simulink model "SWC_HALIN_CDD_type"  (R2021b)
settings: Solver=FixedStepDiscrete  StartTime=0.0  StopTime=10.0  FixedStep=0.005  RelTol=1e-3
values from neighbouring files (symbols this model uses):
  C_TASK_5MS_S = (	C_TICK_TIME_S      	)    [vcu_local_hdr.m]    (also in vcu_local_hdrTA2.m)
  DIDLen_APSFunConfig = uint16(16)    [vcu_local_hdr.m]
  DIDLen_AutoLock = uint16(1)    [vcu_local_hdr.m]
  DIDLen_AutoWipHSpdEN = uint16(1)    [vcu_local_hdr.m]
  DIDLen_DKCKey = uint16(8)    [vcu_local_hdr.m]
  DIDLen_DRLDis = uint16(1)    [vcu_local_hdr.m]
  DIDLen_DynoMode = uint16(1)    [vcu_local_hdr.m]
  DIDLen_FMHTimer = uint16(1)    [vcu_local_hdr.m]
  DIDLen_TireSize = uint16(16)    [vcu_local_hdr.m]
  DIDLen_TurnLampFLThreCurr = uint16(1)    [vcu_local_hdr.m]
  DIDLen_TurnLampFRThreCurr = uint16(1)    [vcu_local_hdr.m]
  DIDLen_TurnLampRLThreCurr = uint16(1)    [vcu_local_hdr.m]
  DIDLen_TurnLampRRThreCurr = uint16(1)    [vcu_local_hdr.m]
  DIDLen_USSConfig = uint16(16)    [vcu_local_hdr.m]
  DIDLen_WipRLSCmdCutFilter = uint16(1)    [vcu_local_hdr.m]
  DIDLen_WipRLSCmdHoldFilter = uint16(1)    [vcu_local_hdr.m]
  DIDLen_XWDMode = uint16(1)    [vcu_local_hdr.m]
  DIDNum_APSFunConfig = uint16(0x0903)    [vcu_local_hdr.m]
  DIDNum_AutoLock = uint16(0x0306)    [vcu_local_hdr.m]
  DIDNum_AutoWipHSpdEN = uint16(0x0308)    [vcu_local_hdr.m]
  DIDNum_DKCKey = uint16(0x0202)    [vcu_local_hdr.m]
  DIDNum_DRLDis = uint16(0x0307)    [vcu_local_hdr.m]
  DIDNum_DynoMode = uint16(0x0203)    [vcu_local_hdr.m]
  DIDNum_FMHTimer = uint16(0x0305)    [vcu_local_hdr.m]
  DIDNum_TireSize = uint16(0x0902)    [vcu_local_hdr.m]
  DIDNum_TurnLampFLThreCurr = uint16(0x0303)    [vcu_local_hdr.m]
  DIDNum_TurnLampFRThreCurr = uint16(0x0301)    [vcu_local_hdr.m]
  DIDNum_TurnLampRLThreCurr = uint16(0x0304)    [vcu_local_hdr.m]
  DIDNum_TurnLampRRThreCurr = uint16(0x0302)    [vcu_local_hdr.m]
  DIDNum_USSConfig = uint16(0x0901)    [vcu_local_hdr.m]
  DIDNum_WipRLSCmdCutFilter = uint16(0x030A)    [vcu_local_hdr.m]
  DIDNum_WipRLSCmdHoldFilter = uint16(0x0309)    [vcu_local_hdr.m]
  DIDNum_XWDMode = uint16(0x0201)    [vcu_local_hdr.m]
  ENUM_DRIVETRAIN_AWD = uint8(  2  )    [vcu_local_hdr.m]
  ENUM_DRIVETRAIN_FWD = uint8(  1  )    [vcu_local_hdr.m]
  ENUM_DRIVETRAIN_RWD = uint8(  0  )    [vcu_local_hdr.m]
  ENUM_REGENLEVEL_LV1 = uint8(  1  )    [vcu_local_hdr.m]
  ENUM_REGENLEVEL_LV2 = uint8(  2  )    [vcu_local_hdr.m]
  ENUM_REGENLEVEL_LV3 = uint8(  3  )    [vcu_local_hdr.m]
  ENUM_REGENLEVEL_LV4 = uint8(  4  )    [vcu_local_hdr.m]
  ENUM_REGENLEVEL_LV5 = uint8(  5  )    [vcu_local_hdr.m]
  ENUM_REGENLEVEL_OPD = uint8(  6  )    [vcu_local_hdr.m]
  ENUM_TPMSSTA_FAT = uint8(  8  )    [vcu_local_hdr.m]
  ENUM_TPMSSTA_LOWBATTERY = uint8(  2  )    [vcu_local_hdr.m]
  ENUM_TPMSSTA_TRIGGER = uint8(  4  )    [vcu_local_hdr.m]
  FALSE = boolean( 0 )    [vcu_local_hdr.m]    (also in vcu_local_hdrTA2.m)
  ONE_INT = uint8(1)    [vcu_local_hdr.m]    (also in vcu_local_hdrTA2.m)
  TRUE = boolean( 1 )    [vcu_local_hdr.m]    (also in vcu_local_hdrTA2.m)
  ZERO_FLOAT = single(0)    [vcu_local_hdr.m]    (also in vcu_local_hdrTA2.m)
  ZERO_INT = uint8(0)    [vcu_local_hdr.m]    (also in vcu_local_hdrTA2.m)
undefined symbols (not defined in the file or in its folder): KHAL_CANBusOffDebounce_s, KHAL_DefaultRegenMode_enum, KHAL_DKCDecryptEnable_flg_ovrdflg, KHAL_DKCDecryptEnable_flg_ovrdval, KHAL_RandomNumberY1_enum, KHAL_RandomNumberY2_enum, KHAL_RandomNumberY_ovrdflg, KHAL_TPMSRESBUTT_flg_ovrdflg, KHAL_TPMSRESBUTT_flg_ovrdval, KINP_ReadVinCode_flg, R_NVMReadCDD_Inner_NVM_ReadOperation
libraries: simulink x112, hcu_lib x23, hdlsllib x8
(part 1 of 7)
settings Model: DataDictionary=APPTypes.sldd  Creator=FVT22063  LastModifiedBy=FVT23033
settings DataIOCC: SaveFormat=StructureWithTime
settings OptimizationCC: DefaultParameterBehavior=Inlined  EnhancedBackFolding=on  PassReuseOutputArgsAs=Individual arguments  ZeroExternalMemoryAtStartup=off  ZeroInternalMemoryAtStartup=off  OptimizeBlockOrder=speed  DifferentSizesBufferReuse=on  OptimizationCustomize=off  EfficientTunableParamExpr=on
settings DebuggingCC: ParameterTunabilityLossMsg=error
settings HardwareCC: ProdBitPerPointer=32  ProdBitPerSizeT=32  ProdBitPerPtrDiffT=32  ProdLargestAtomicInteger=Long  ProdLargestAtomicFloat=Double  ProdWordSize=32  ProdLongLongMode=on  ProdHWDeviceType=ARM Compatible->ARM Cortex-M
settings ModelReferenceCC: ModelReferenceNumInstancesAllowed=Single
settings SFSimCC: MATLABDynamicMemAlloc=off
settings RTWCC: Description=AUTOSAR  SystemTargetFile=autosar.tlc  GenCodeOnly=on  TemplateMakefile=ert_default_tmf  PortableWordSizes=on
settings CodeAppCC: ForceParamTrailComments=on  IgnoreCustomStorageClasses=off  OperatorAnnotations=on  SimulinkDataObjDesc=on  SFDataObjDesc=on  InsertBlockDesc=on
settings STFCustomTargetCC: TargetLangStandard=C99 (ISO)  MultiwordLength=256  ParMdlRefBuildCompliant=on  CompOptLevelCompliant=on  IncludeMdlTerminateFcn=off  CombineOutputUpdateFcns=on  SuppressErrorStatus=on  ERTCustomFileBanners=on  SupportNonFinite=off  SupportComplex=off  SupportContinuousTime=off  SupportNonInlinedSFcns=off  RemoveResetFunc=on  MATLABClassNameForMDSCustomization=Simulink.SoftwareTarget.ERTCustomization  AutosarCompliant=on  GRTInterface=off  UseToolchainInfoCompliant=on  LookupTableObjectStructAxisOrder=2,1,3,4,...  LUTObjectStructOrderEvenSpacing=Size,Table,Breakpoints  SystemTargetFile=autosar.tlc
settings ERTTargetCC: TargetLangStandard=C99 (ISO)  ConcurrentExecutionCompliant=off  IncludeMdlTerminateFcn=off  SuppressErrorStatus=on  SupportNonFinite=off  SupportComplex=off  ModelStepFunctionPrototypeControlCompliant=off  CPPClassGenCompliant=off  AutosarCompliant=on  LookupTableObjectStructAxisOrder=2,1,3,4,...  LUTObjectStructOrderEvenSpacing=Size,Table,Breakpoints  GenerateASAP2=on  InlinedParameterPlacement=NonHierarchical  ERTCustomFileTemplate=example_file_process.tlc  ConvertIfToSwitch=off  SuppressUnreachableDefaultCases=off  BooleanTrueId=true_MatlabRTW  BooleanFalseId=false_MatlabRTW

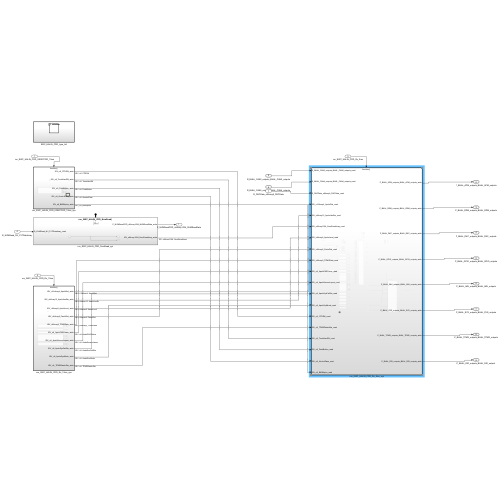
[thumbnail: Simulink's stored preview of the top-level diagram]
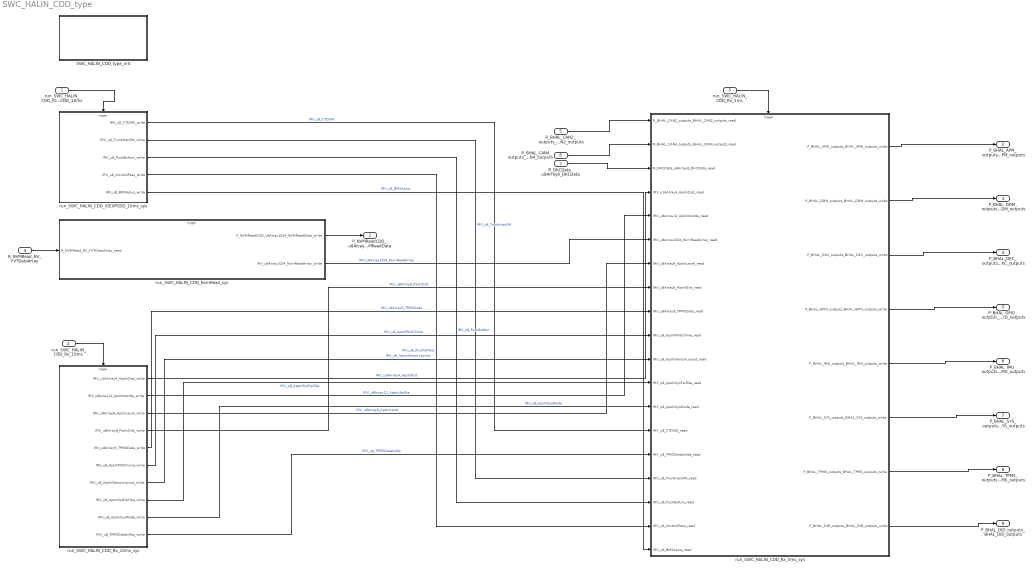
== system SWC_HALIN_CDD_type ==
  run_SWC_HALIN_CDD_IOEXPCDD_10ms : Inport  SampleTime=0.01  OutputFunctionCall=on
  run_SWC_HALIN_CDD_Rx_10ms : Inport  Port=2  SampleTime=0.01  OutputFunctionCall=on
  run_SWC_HALIN_CDD_Rx_5ms : Inport  Port=3  SampleTime=0.005  OutputFunctionCall=on
  R_NVMRead_NV_FVTDataArray : Inport  Port=4  OutDataTypeStr=uint8  PortDimensions=1024
  R_BHAL_CAN2_outputs_BHAL_CAN2_outputs : Inport  Port=5  OutDataTypeStr=Bus: BHAL_CAN2_outputs  PortDimensions=1  BusOutputAsStruct=on
  R_BHAL_CAN4_outputs_BHAL_CAN4_outputs : Inport  Port=6  OutDataTypeStr=Bus: BHAL_CAN4_outputs  PortDimensions=1  BusOutputAsStruct=on
  R_DKCData_u8Array8_DKCData : Inport  Port=7  OutDataTypeStr=uint8  PortDimensions=8
  SWC_HALIN_CDD_type_Init : Subsystem
  run_SWC_HALIN_CDD_IOEXPCDD_10ms_sys : Subsystem
  run_SWC_HALIN_CDD_NvmRead_sys : Subsystem
  run_SWC_HALIN_CDD_Rx_10ms_sys : Subsystem
  run_SWC_HALIN_CDD_Rx_5ms_sys : Subsystem
  P_NVMReadCDD_u8Array1024_NVMReadData : Outport  OutDataTypeStr=uint8  PortDimensions=1024
  P_BHAL_APM_outputs_BHAL_APM_outputs : Outport  Port=2  OutDataTypeStr=Bus: BHAL_APM_outputs  PortDimensions=1  BusOutputAsStruct=on
  P_BHAL_DDM_outputs_BHAL_DDM_outputs : Outport  Port=3  OutDataTypeStr=Bus: BHAL_DDM_outputs  PortDimensions=1  BusOutputAsStruct=on
  P_BHAL_DKC_outputs_BHAL_DKC_outputs : Outport  Port=4  OutDataTypeStr=Bus: BHAL_DKC_outputs  PortDimensions=1  BusOutputAsStruct=on
  P_BHAL_GPIO_outputs_BHAL_GPIO_outputs : Outport  Port=5  OutDataTypeStr=Bus: BHAL_GPIO_outputs  PortDimensions=1  BusOutputAsStruct=on
  P_BHAL_IMU_outputs_BHAL_IMU_outputs : Outport  Port=6  OutDataTypeStr=Bus: BHAL_IMU_outputs  PortDimensions=1  BusOutputAsStruct=on
  P_BHAL_SYS_outputs_BHAL_SYS_outputs : Outport  Port=7  OutDataTypeStr=Bus: BHAL_SYS_outputs  PortDimensions=1  BusOutputAsStruct=on
  P_BHAL_TPMS_outputs_BHAL_TPMS_outputs : Outport  Port=8  OutDataTypeStr=Bus: BHAL_TPMS_outputs  PortDimensions=1  BusOutputAsStruct=on
  P_BHAL_DID_outputs_BHAL_DID_outputs : Outport  Port=9  OutDataTypeStr=Bus: BHAL_DID_outputs  PortDimensions=1  BusOutputAsStruct=on
  wires:
  R_NVMRead_NV_FVTDataArray/1 -> run_SWC_HALIN_CDD_NvmRead_sys/1(R_NVMRead_NV_FVTDataArray_read)
  run_SWC_HALIN_CDD_NvmRead_sys/1(P_NVMReadCDD_u8Array1024_NVMReadData_write) -> P_NVMReadCDD_u8Array1024_NVMReadData/1
  R_BHAL_CAN2_outputs_BHAL_CAN2_outputs/1 -> run_SWC_HALIN_CDD_Rx_5ms_sys/1(R_BHAL_CAN2_outputs_BHAL_CAN2_outputs_read)
  R_BHAL_CAN4_outputs_BHAL_CAN4_outputs/1 -> run_SWC_HALIN_CDD_Rx_5ms_sys/2(R_BHAL_CAN4_outputs_BHAL_CAN4_outputs_read)
  R_DKCData_u8Array8_DKCData/1 -> run_SWC_HALIN_CDD_Rx_5ms_sys/3(R_DKCData_u8Array8_DKCData_read)
  run_SWC_HALIN_CDD_Rx_5ms_sys/1(P_BHAL_APM_outputs_BHAL_APM_outputs_write) -> P_BHAL_APM_outputs_BHAL_APM_outputs/1
  run_SWC_HALIN_CDD_Rx_5ms_sys/2(P_BHAL_DDM_outputs_BHAL_DDM_outputs_write) -> P_BHAL_DDM_outputs_BHAL_DDM_outputs/1
  run_SWC_HALIN_CDD_Rx_5ms_sys/3(P_BHAL_DKC_outputs_BHAL_DKC_outputs_write) -> P_BHAL_DKC_outputs_BHAL_DKC_outputs/1
  run_SWC_HALIN_CDD_Rx_5ms_sys/4(P_BHAL_GPIO_outputs_BHAL_GPIO_outputs_write) -> P_BHAL_GPIO_outputs_BHAL_GPIO_outputs/1
  run_SWC_HALIN_CDD_Rx_5ms_sys/5(P_BHAL_IMU_outputs_BHAL_IMU_outputs_write) -> P_BHAL_IMU_outputs_BHAL_IMU_outputs/1
  run_SWC_HALIN_CDD_Rx_5ms_sys/6(P_BHAL_SYS_outputs_BHAL_SYS_outputs_write) -> P_BHAL_SYS_outputs_BHAL_SYS_outputs/1
  run_SWC_HALIN_CDD_Rx_5ms_sys/7(P_BHAL_TPMS_outputs_BHAL_TPMS_outputs_write) -> P_BHAL_TPMS_outputs_BHAL_TPMS_outputs/1
  run_SWC_HALIN_CDD_Rx_5ms_sys/8(P_BHAL_DID_outputs_BHAL_DID_outputs_write) -> P_BHAL_DID_outputs_BHAL_DID_outputs/1
  run_SWC_HALIN_CDD_IOEXPCDD_10ms_sys/1(IRV_u8_CTDSW_write) -> run_SWC_HALIN_CDD_Rx_5ms_sys/14(IRV_u8_CTDSW_read)  "IRV_u8_CTDSW"
  run_SWC_HALIN_CDD_IOEXPCDD_10ms_sys/2(IRV_u8_TrunkHanSW_write) -> run_SWC_HALIN_CDD_Rx_5ms_sys/16(IRV_u8_TrunkHanSW_read)  "IRV_u8_TrunkHanSW"
  run_SWC_HALIN_CDD_IOEXPCDD_10ms_sys/3(IRV_u8_PushButton_write) -> run_SWC_HALIN_CDD_Rx_5ms_sys/17(IRV_u8_PushButton_read)  "IRV_u8_PushButton"
  run_SWC_HALIN_CDD_IOEXPCDD_10ms_sys/4(IRV_u8_AlcoholPass_write) -> run_SWC_HALIN_CDD_Rx_5ms_sys/18(IRV_u8_AlcoholPass_read)  "IRV_u8_AlcoholPass"
  run_SWC_HALIN_CDD_NvmRead_sys/2(IRV_u8Array1024_NvmReadArray_write) -> run_SWC_HALIN_CDD_Rx_5ms_sys/6(IRV_u8Array1024_NvmReadArray_read)  "IRV_u8Array1024_NvmReadArray"
  run_SWC_HALIN_CDD_Rx_10ms_sys/1(IRV_u16Array4_ApsInDist_write) -> run_SWC_HALIN_CDD_Rx_5ms_sys/4(IRV_u16Array4_ApsInDist_read)  "IRV_u16Array4_ApsInDist"
  run_SWC_HALIN_CDD_Rx_10ms_sys/2(IRV_u8Array12_ApsInUssSta_write) -> run_SWC_HALIN_CDD_Rx_5ms_sys/5(IRV_u8Array12_ApsInUssSta_read)  "IRV_u8Array12_ApsInUssSta"
  run_SWC_HALIN_CDD_Rx_10ms_sys/3(IRV_u8Array8_ApsInLevel_write) -> run_SWC_HALIN_CDD_Rx_5ms_sys/7(IRV_u8Array8_ApsInLevel_read)  "IRV_u8Array8_ApsInLevel"
  run_SWC_HALIN_CDD_Rx_10ms_sys/4(IRV_u8Array8_PasInDist_write) -> run_SWC_HALIN_CDD_Rx_5ms_sys/8(IRV_u8Array8_PasInDist_read)  "IRV_u8Array8_PasInDist"
  run_SWC_HALIN_CDD_Rx_10ms_sys/5(IRV_u8Array9_TPMSData_write) -> run_SWC_HALIN_CDD_Rx_5ms_sys/9(IRV_u8Array9_TPMSData_read)  "IRV_u8Array9_TPMSData"
  run_SWC_HALIN_CDD_Rx_10ms_sys/6(IRV_u8_ApsInPASChime_write) -> run_SWC_HALIN_CDD_Rx_5ms_sys/10(IRV_u8_ApsInPASChime_read)  "IRV_u8_ApsInPASChime"
  run_SWC_HALIN_CDD_Rx_10ms_sys/7(IRV_u8_ApsInSensorLayout_write) -> run_SWC_HALIN_CDD_Rx_5ms_sys/11(IRV_u8_ApsInSensorLayout_read)  "IRV_u8_ApsInSensorLayout"
  run_SWC_HALIN_CDD_Rx_10ms_sys/8(IRV_u8_ApsInSysFailSta_write) -> run_SWC_HALIN_CDD_Rx_5ms_sys/12(IRV_u8_ApsInSysFailSta_read)  "IRV_u8_ApsInSysFailSta"
  run_SWC_HALIN_CDD_Rx_10ms_sys/9(IRV_u8_ApsInSysMode_write) -> run_SWC_HALIN_CDD_Rx_5ms_sys/13(IRV_u8_ApsInSysMode_read)  "IRV_u8_ApsInSysMode"
  run_SWC_HALIN_CDD_Rx_10ms_sys/10(IRV_u8_TPMSDataInSta_write) -> run_SWC_HALIN_CDD_Rx_5ms_sys/15(IRV_u8_TPMSDataInSta_read)  "IRV_u8_TPMSDataInSta"
  run_SWC_HALIN_CDD_IOEXPCDD_10ms/1 -> run_SWC_HALIN_CDD_IOEXPCDD_10ms_sys/Trigger
  run_SWC_HALIN_CDD_Rx_10ms/1 -> run_SWC_HALIN_CDD_Rx_10ms_sys/Trigger
  run_SWC_HALIN_CDD_Rx_5ms/1 -> run_SWC_HALIN_CDD_Rx_5ms_sys/Trigger
  run_SWC_HALIN_CDD_IOEXPCDD_10ms_sys/5(IRV_u8_BMSAplus_write) -> run_SWC_HALIN_CDD_Rx_5ms_sys/19(IRV_u8_BMSAplus_read)  "IRV_u8_BMSAplus"

== system SWC_HALIN_CDD_type/SWC_HALIN_CDD_type_Init ==
  Event Listener : EventListener  EventName=reset

== system SWC_HALIN_CDD_type/run_SWC_HALIN_CDD_IOEXPCDD_10ms_sys ==
  function : TriggerPort  TriggerType=function-call  VariantControl=(inherit)  SampleTimeType=periodic  SampleTime=-1
  R_IOExpIN_CDD_CSOP_IOExpGetVal : FunctionCaller  FunctionPrototype=[u8_CTDSW,u8_TrunkHanSW,u8_PushButton,u8_AlcoholPass,u8_BMSAplus] = R_IOExpIN_CDD_CSOP_IOExpGetVal()  OutputArgumentSpecifications=uint8(1), uint8(1), uint8(1), uint8(1), uint8(1)
  IRV_u8_CTDSW_write : Outport  OutDataTypeStr=uint8  PortDimensions=1
  IRV_u8_TrunkHanSW_write : Outport  Port=2  OutDataTypeStr=uint8  PortDimensions=1
  IRV_u8_PushButton_write : Outport  Port=3  OutDataTypeStr=uint8  PortDimensions=1
  IRV_u8_AlcoholPass_write : Outport  Port=4  OutDataTypeStr=uint8  PortDimensions=1
  IRV_u8_BMSAplus_write : Outport  Port=5  OutDataTypeStr=uint8  PortDimensions=1
  wires:
  R_IOExpIN_CDD_CSOP_IOExpGetVal/1 -> IRV_u8_CTDSW_write/1
  R_IOExpIN_CDD_CSOP_IOExpGetVal/2 -> IRV_u8_TrunkHanSW_write/1
  R_IOExpIN_CDD_CSOP_IOExpGetVal/3 -> IRV_u8_PushButton_write/1
  R_IOExpIN_CDD_CSOP_IOExpGetVal/4 -> IRV_u8_AlcoholPass_write/1
  R_IOExpIN_CDD_CSOP_IOExpGetVal/5 -> IRV_u8_BMSAplus_write/1

== system SWC_HALIN_CDD_type/run_SWC_HALIN_CDD_NvmRead_sys ==
  R_NVMRead_NV_FVTDataArray_read : Inport
  function : TriggerPort  TriggerType=function-call  IsSimulinkFunction=on  FunctionName=run_SWC_HALIN_CDD_NvmRead  VariantControl=(inherit)
  P_NVMReadCDD_u8Array1024_NVMReadData_write : Outport
  IRV_u8Array1024_NvmReadArray_write : Outport  Port=2  OutDataTypeStr=uint8  PortDimensions=1024
  wires:
  R_NVMRead_NV_FVTDataArray_read/1 -> IRV_u8Array1024_NvmReadArray_write/1, P_NVMReadCDD_u8Array1024_NVMReadData_write/1

== system SWC_HALIN_CDD_type/run_SWC_HALIN_CDD_Rx_10ms_sys ==
  function : TriggerPort  TriggerType=function-call  VariantControl=(inherit)  SampleTimeType=periodic  SampleTime=-1
  R_HALINCDD_CSOP_TPMS_GetRawData : FunctionCaller  FunctionPrototype=[u8_TPMSDataInSta,u8Array9_TPMSData] = R_HALINCDD_CSOP_TPMS_GetRawData()  OutputArgumentSpecifications=boolean(true), uint8([1;1;1;1;1;1;1;1;1])
  R_HALIN_APS_CSOP_ApsGetDist : FunctionCaller  FunctionPrototype=[u8Array8_PasInDist,u16Array4_ApsInDist] = R_HALIN_APS_CSOP_ApsGetDist()  OutputArgumentSpecifications=uint8([1;1;1;1;1;1;1;1]), uint16([1;1;1;1])
  R_HALIN_APS_CSOP_ApsGetDistLevel : FunctionCaller  FunctionPrototype=u8Array8_ApsInLevel = R_HALIN_APS_CSOP_ApsGetDistLevel()  OutputArgumentSpecifications=uint8([1;1;1;1;1;1;1;1])
  R_HALIN_APS_CSOP_ApsGetOtherStatus : FunctionCaller  FunctionPrototype=[u8_ApsInPASChime,u8_ApsInSensorLayout,u8_ApsInSysFailSta,u8_ApsInSysMode] = R_HALIN_APS_CSOP_ApsGetOtherStatus()  OutputArgumentSpecifications=uint8(1), uint8(1), uint8(1), uint8(1)
  R_HALIN_APS_CSOP_ApsGetUssSta : FunctionCaller  FunctionPrototype=u8Array12_ApsInUssSta = R_HALIN_APS_CSOP_ApsGetUssSta()  OutputArgumentSpecifications=uint8([1;1;1;1;1;1;1;1;1;1;1;1])
  IRV_u16Array4_ApsInDist_write : Outport  OutDataTypeStr=uint16  PortDimensions=4
  IRV_u8Array12_ApsInUssSta_write : Outport  Port=2  OutDataTypeStr=uint8  PortDimensions=12
  IRV_u8Array8_ApsInLevel_write : Outport  Port=3  OutDataTypeStr=uint8  PortDimensions=8
  IRV_u8Array8_PasInDist_write : Outport  Port=4  OutDataTypeStr=uint8  PortDimensions=8
  IRV_u8Array9_TPMSData_write : Outport  Port=5  OutDataTypeStr=uint8  PortDimensions=9
  IRV_u8_ApsInPASChime_write : Outport  Port=6  OutDataTypeStr=uint8  PortDimensions=1
  IRV_u8_ApsInSensorLayout_write : Outport  Port=7  OutDataTypeStr=uint8  PortDimensions=1
  IRV_u8_ApsInSysFailSta_write : Outport  Port=8  OutDataTypeStr=uint8  PortDimensions=1
  IRV_u8_ApsInSysMode_write : Outport  Port=9  OutDataTypeStr=uint8  PortDimensions=1
  IRV_u8_TPMSDataInSta_write : Outport  Port=10  OutDataTypeStr=boolean  PortDimensions=1
  wires:
  R_HALIN_APS_CSOP_ApsGetDist/1 -> IRV_u8Array8_PasInDist_write/1
  R_HALIN_APS_CSOP_ApsGetDist/2 -> IRV_u16Array4_ApsInDist_write/1
  R_HALIN_APS_CSOP_ApsGetDistLevel/1 -> IRV_u8Array8_ApsInLevel_write/1
  R_HALIN_APS_CSOP_ApsGetUssSta/1 -> IRV_u8Array12_ApsInUssSta_write/1
  R_HALIN_APS_CSOP_ApsGetOtherStatus/1 -> IRV_u8_ApsInPASChime_write/1
  R_HALIN_APS_CSOP_ApsGetOtherStatus/2 -> IRV_u8_ApsInSensorLayout_write/1
  R_HALIN_APS_CSOP_ApsGetOtherStatus/3 -> IRV_u8_ApsInSysFailSta_write/1
  R_HALIN_APS_CSOP_ApsGetOtherStatus/4 -> IRV_u8_ApsInSysMode_write/1
  R_HALINCDD_CSOP_TPMS_GetRawData/1 -> IRV_u8_TPMSDataInSta_write/1
  R_HALINCDD_CSOP_TPMS_GetRawData/2 -> IRV_u8Array9_TPMSData_write/1

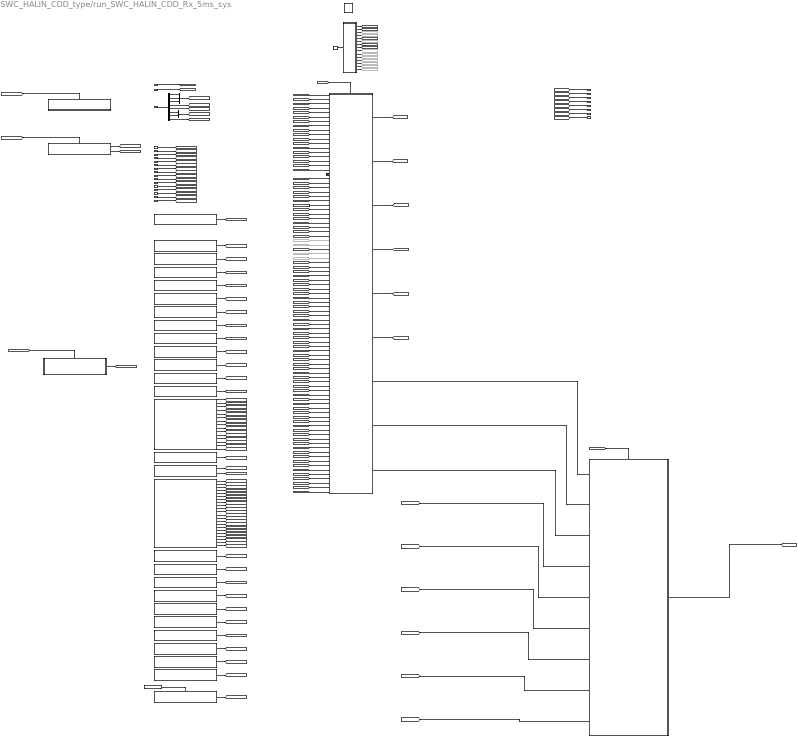
== system SWC_HALIN_CDD_type/run_SWC_HALIN_CDD_Rx_5ms_sys ==
  R_BHAL_CAN2_outputs_BHAL_CAN2_outputs_read : Inport
  R_BHAL_CAN4_outputs_BHAL_CAN4_outputs_read : Inport  Port=2
  R_DKCData_u8Array8_DKCData_read : Inport  Port=3
  IRV_u16Array4_ApsInDist_read : Inport  Port=4
  IRV_u8Array12_ApsInUssSta_read : Inport  Port=5
  IRV_u8Array1024_NvmReadArray_read : Inport  Port=6
  IRV_u8Array8_ApsInLevel_read : Inport  Port=7
  IRV_u8Array8_PasInDist_read : Inport  Port=8
  IRV_u8Array9_TPMSData_read : Inport  Port=9
  IRV_u8_ApsInPASChime_read : Inport  Port=10
  IRV_u8_ApsInSensorLayout_read : Inport  Port=11
  IRV_u8_ApsInSysFailSta_read : Inport  Port=12
  IRV_u8_ApsInSysMode_read : Inport  Port=13
  IRV_u8_CTDSW_read : Inport  Port=14
  IRV_u8_TPMSDataInSta_read : Inport  Port=15
  IRV_u8_TrunkHanSW_read : Inport  Port=16
  IRV_u8_PushButton_read : Inport  Port=17
  IRV_u8_AlcoholPass_read : Inport  Port=18
  IRV_u8_BMSAplus_read : Inport  Port=19
  function : TriggerPort  TriggerType=function-call  VariantControl=(inherit)  SampleTimeType=periodic  SampleTime=-1
  Constant5 : Constant  Value=FALSE
  Constant6 : Constant  Value=ONE_INT
  Constant8 : Constant  Value=KINP_ReadVinCode_flg
  DIDGet_Subsystem : Subsystem
  Demux : Demux  Outputs=8
  From91 : From  Commented=on  GotoTag=u8_DidStaXWD
  From92 : From  Commented=on  GotoTag=u8Array8_DidDataDKC
  From96 : From  Commented=on  GotoTag=u8_DidDataXWD
  From97 : From  Commented=on  GotoTag=u8_DidStaDKC
  Goto101 : Goto  Commented=on  GotoTag=trig_HAL_OUTAFTER_50_1
  Goto106 : Goto  Commented=on  GotoTag=trig_GetNMID
  Goto119 : Goto  Commented=on  GotoTag=trig_HAL_DKC_10_3
  Goto91 : Goto  Commented=on  GotoTag=trig_WDG
  Goto94 : Goto  Commented=on  GotoTag=trig_HAL_OUT_50
  Goto95 : Goto  Commented=on  GotoTag=trig_OUTP_AFTER_40_1
  Goto96 : Goto  Commented=on  GotoTag=trig_OUTP_40
  Goto97 : Goto  Commented=on  GotoTag=trig_APP_30
  Goto98 : Goto  Commented=on  GotoTag=trig_INP_20
  Goto99 : Goto  Commented=on  GotoTag=trig_HAL_IN_10
  Ground_1 : Ground
  Halin_CDD : Subsystem
      settings: RTWSystemCode=Nonreusable function  RTWFcnNameOpts=Use subsystem name  RTWFileNameOpts=Use subsystem name
  Mux : Mux  Inputs=3
  Mux1 : Mux  Inputs=2
  R_HALINCDD_CSOP_AnyNmID : FunctionCaller  FunctionPrototype=u8_AnyNMID = R_HALINCDD_CSOP_AnyNmID()  OutputArgumentSpecifications=uint8(1)
  R_HALINCDD_CSOP_CAN1BusOff : FunctionCaller  FunctionPrototype=u8_CAN1BusOff = R_HALINCDD_CSOP_CAN1BusOff()  OutputArgumentSpecifications=uint8(1)
  R_HALINCDD_CSOP_CAN2BusOff : FunctionCaller  FunctionPrototype=u8_CAN2BusOff = R_HALINCDD_CSOP_CAN2BusOff()  OutputArgumentSpecifications=uint8(1)
  R_HALINCDD_CSOP_CAN3BusOff : FunctionCaller  FunctionPrototype=u8_CAN3BusOff = R_HALINCDD_CSOP_CAN3BusOff()  OutputArgumentSpecifications=uint8(1)
  R_HALINCDD_CSOP_CAN4BusOff : FunctionCaller  FunctionPrototype=u8_CAN4BusOff = R_HALINCDD_CSOP_CAN4BusOff()  OutputArgumentSpecifications=uint8(1)
  R_HALINCDD_CSOP_CAN5BusOff : FunctionCaller  FunctionPrototype=u8_CAN5BusOff = R_HALINCDD_CSOP_CAN5BusOff()  OutputArgumentSpecifications=uint8(1)
  R_HALINCDD_CSOP_CAN6BusOff : FunctionCaller  FunctionPrototype=u8_CAN6BusOff = R_HALINCDD_CSOP_CAN6BusOff()  OutputArgumentSpecifications=uint8(1)
  R_HALINCDD_CSOP_GetAcoreReadyToSleep : FunctionCaller  FunctionPrototype=s8_AcoreReadyToSleep = R_HALINCDD_CSOP_GetAcoreReadyToSleep()  OutputArgumentSpecifications=int8(1)
  R_HALINCDD_CSOP_GetAcoreRebootCmd : FunctionCaller  FunctionPrototype=u8_AcoreRebootCmd = R_HALINCDD_CSOP_GetAcoreRebootCmd()  OutputArgumentSpecifications=uint8(1)
  R_HALINCDD_CSOP_GetAuxBattVoltage : FunctionCaller  FunctionPrototype=u16_AuxBattVol100mV = R_HALINCDD_CSOP_GetAuxBattVoltage()  OutputArgumentSpecifications=uint16(1)
  R_HALINCDD_CSOP_GetBootPath : FunctionCaller  FunctionPrototype=u32_BootPath = R_HALINCDD_CSOP_GetBootPath()  OutputArgumentSpecifications=uint32(1)
  R_HALINCDD_CSOP_GetBootReason : FunctionCaller  FunctionPrototype=u8_BootReason = R_HALINCDD_CSOP_GetBootReason()  OutputArgumentSpecifications=uint8(1)
  R_HALINCDD_CSOP_GetEvccAplusPwrUpReq : FunctionCaller  FunctionPrototype=u8_EvccAplusPwrUpReq = R_HALINCDD_CSOP_GetEvccAplusPwrUpReq()  OutputArgumentSpecifications=uint8(1)
  R_HALINCDD_CSOP_GetNmState : FunctionCaller  FunctionPrototype=u8_CurrentNMState = R_HALINCDD_CSOP_GetNmState()  OutputArgumentSpecifications=uint8(1)
  R_HALINCDD_CSOP_GetNvmProtectState : FunctionCaller  FunctionPrototype=u8_NvmProtectSta = R_HALINCDD_CSOP_GetNvmProtectState()  OutputArgumentSpecifications=uint8(1)
  R_HALINCDD_CSOP_GetSWID : FunctionCaller  FunctionPrototype=u8Array33_SWID = R_HALINCDD_CSOP_GetSWID()  OutputArgumentSpecifications=uint8([1;1;1;1;1;1;1;1;1;1;1;1;1;1;1;1;1;1;1;1;1;1;1;1;1;1;1;1;1;1;1;1;1])
  R_HALINCDD_CSOP_GetVinCode : Subsystem
  R_HALINCDD_CSOP_GetVinpAllowMoveThdOta : FunctionCaller  FunctionPrototype=u8_AllowMovThdOTA = R_HALINCDD_CSOP_GetVinpAllowMoveThdOta()  OutputArgumentSpecifications=uint8(1)
  R_HALINCDD_CSOP_GetVinpPwrReqOta : FunctionCaller  FunctionPrototype=u8_PwrReqOTA = R_HALINCDD_CSOP_GetVinpPwrReqOta()  OutputArgumentSpecifications=uint8(1)
  R_HALINCDD_CSOP_GetWISR : FunctionCaller  FunctionPrototype=u32_WISR = R_HALINCDD_CSOP_GetWISR()  OutputArgumentSpecifications=uint32(1)
  R_HALINCDD_CSOP_HALINCDD_DIRECT : FunctionCaller  FunctionPrototype=[u8_BrakeSW,u8_BrakeLamp,f32_Pedal1Vol,f32_Pedal2Vol,f32_Pedal1Ref5V,f32_Pedal2Ref5V,u8_DrDoorSW,u8_PsDoorSW,u8_RRDoorSW,u8_RLDoorSW,u8_HoodSW,u8_TailgateSW,u8_HazardSW,u8_SeatSW,u8_CrashSignal] = R_HALINCDD_CSOP_HALINCDD_DIRECT()  OutputArgumentSpecifications=uint8(1), uint8(1), single(1), single(1), single(1), single(1), uint8(1), uint8(1), uint8(1), uint8(1), uint8(1), uint8(1), uint8(1), uint8(1), uint8(1)
  R_HALINCDD_CSOP_ReadPedalZeroPosReq : FunctionCaller  FunctionPrototype=u8_ReadPedalZeroPosReq = R_HALINCDD_CSOP_ReadPedalZeroPosReq()  OutputArgumentSpecifications=uint8(1)
  R_HALINCDD_CSOP_ResetPedalZeroPosReq : FunctionCaller  FunctionPrototype=u8_ResetPedalZeroPosReq = R_HALINCDD_CSOP_ResetPedalZeroPosReq()  OutputArgumentSpecifications=uint8(1)
  R_HALINCDD_CSOP_TPMSSensorIDRegGetSta : FunctionCaller  FunctionPrototype=u8_TPMSSensorIDRegSta = R_HALINCDD_CSOP_TPMSSensorIDRegGetSta()  OutputArgumentSpecifications=uint8(1)
  R_HALINCDD_u8Array4_HWID : FunctionCaller  FunctionPrototype=u8Array4_HWID = R_HALINCDD_u8Array4_HWID()  OutputArgumentSpecifications=uint8([1;1;1;1])
  R_HALIN_APS_CSOP_ApsGetData : FunctionCaller  FunctionPrototype=[u8_GetAPS_Progress_PCT,u8_GetAPS_RQ_Display,u8_GetAPS_SW_Ver,u8_GetAPS_HW_Ver,u8_GetAPS_ExitCondition,f32_GetAPS_Angle_Target,u8_GetAPS_Sta_System,u8_GetAPS_V_Rq_EPAS_Ctrl,u8_GetAPS_Rq_EPAS_Ctrl,u8_GetAPS_Req,f32_GetAPS_DecReq,u8_GetAPS_DecReq_A,f32_GetAPS_SpeedCmd,u8_GetAPS_ShftPosnReq,u8_GetAPS_VMC_Req_A,u8_GetCAAS_Sta,u8_GetCAAS_VMC_Req_A,u8_GetAPS_PwrReq_cmd,u8_GetRAPS_BCM_LockReq_Cmd,u8_GetRAPS_BCM_Lamp_Cmd,u8_GetRAPS_ErrWarn_Sta,u8_GetRAPS_ErrLv1_flg] = R_HALIN_APS_CSOP_ApsGetData()  OutputArgumentSpecifications=uint8(1), uint8(1), uint8(1), uint8(1), uint8(1), single(1), uint8(1), uint8(1), uint8(1), uint8(1), single(1), uint8(1), single(1), uint8(1), uint8(1), uint8(1), uint8(1), uint8(1), uint8(1), uint8(1), uint8(1), uint8(1)
  R_HALIN_IMU_CSOP_IMUGetOffsetVal : Subsystem
  R_HALIN_IMU_CSOP_IMUGetSixAxisVal : FunctionCaller  FunctionPrototype=[s16_IMUSixAxisVal,u8_IMUSixAxisValSta] = R_HALIN_IMU_CSOP_IMUGetSixAxisVal()  OutputArgumentSpecifications=int16([1;1;1;1;1;1]), uint8(1)
  R_NVMReadCDD_Inner_NVM_ReadOperation : Subsystem
  R_UDSCDD_CSOP_DdmClearDTCNotification : FunctionCaller  FunctionPrototype=u8_ClearDTCcmd = R_UDSCDD_CSOP_DdmClearDTCNotification()  OutputArgumentSpecifications=uint8(1)
  Subsystem : Subsystem
  hcu_main_sched : Stateflow chart  TreatAsAtomicUnit=on
  P_BHAL_APM_outputs_BHAL_APM_outputs_write : Outport
  P_BHAL_DDM_outputs_BHAL_DDM_outputs_write : Outport  Port=2
  P_BHAL_DKC_outputs_BHAL_DKC_outputs_write : Outport  Port=3
  P_BHAL_GPIO_outputs_BHAL_GPIO_outputs_write : Outport  Port=4
  P_BHAL_IMU_outputs_BHAL_IMU_outputs_write : Outport  Port=5
  P_BHAL_SYS_outputs_BHAL_SYS_outputs_write : Outport  Port=6
  P_BHAL_TPMS_outputs_BHAL_TPMS_outputs_write : Outport  Port=7
  P_BHAL_DID_outputs_BHAL_DID_outputs_write : Outport  Port=8
  wires:
  IRV_u16Array4_ApsInDist_read/1 -> [u16Array4_ApsInDist]
  IRV_u8Array12_ApsInUssSta_read/1 -> [u8Array12_ApsInUssSta]
  IRV_u8Array1024_NvmReadArray_read/1 -> [u8Array1024_NvmReadArray]
  IRV_u8Array8_ApsInLevel_read/1 -> [u8Array8_ApsInLevel]
  IRV_u8Array8_PasInDist_read/1 -> [u8Array8_PasInDist]
  IRV_u8Array9_TPMSData_read/1 -> [u8Array9_TPMSData]
  IRV_u8_ApsInPASChime_read/1 -> [u8_ApsInPASChime]
  IRV_u8_ApsInSensorLayout_read/1 -> [u8_ApsInSensorLayout]
  IRV_u8_ApsInSysFailSta_read/1 -> [u8_ApsInSysFailSta]
  IRV_u8_ApsInSysMode_read/1 -> [u8_ApsInSysMode]
  IRV_u8_CTDSW_read/1 -> [u8_CTDSW]
  IRV_u8_TPMSDataInSta_read/1 -> [u8_TPMSDataInSta]
  IRV_u8_TrunkHanSW_read/1 -> [u8_TrunkHanSW]
  IRV_u8_PushButton_read/1 -> [u8_PushButton]
  IRV_u8_AlcoholPass_read/1 -> [u8_AlcoholPass]
  R_HALINCDD_CSOP_AnyNmID/1 -> [u8_AnyNMID]
  R_HALINCDD_CSOP_GetAcoreReadyToSleep/1 -> [s8_AcoreReadyToSleep]
  R_HALINCDD_CSOP_GetAuxBattVoltage/1 -> [u16_AuxBattVol100mV]
  R_HALINCDD_CSOP_GetBootReason/1 -> [u8_BootReason]
  R_HALINCDD_CSOP_GetBootPath/1 -> [u32_BootPath]
  R_HALINCDD_CSOP_GetEvccAplusPwrUpReq/1 -> [u8_EvccAplusPwrUpReq]
  R_HALINCDD_u8Array4_HWID/1 -> [u8Array4_HWID]
  R_HALINCDD_CSOP_GetNvmProtectState/1 -> [u8_NvmProtectSta]
  R_HALINCDD_CSOP_GetNmState/1 -> [u8_CurrentNMState]
  R_HALINCDD_CSOP_GetSWID/1 -> [u8Array33_SWID]
  R_HALINCDD_CSOP_GetVinpAllowMoveThdOta/1 -> [u8_AllowMovThdOTA]
  R_HALINCDD_CSOP_GetVinpPwrReqOta/1 -> [u8_PwrReqOTA]
  R_HALINCDD_CSOP_GetWISR/1 -> [u32_WISR]
  R_HALINCDD_CSOP_HALINCDD_DIRECT/1 -> [u8_BrakeSW]
  R_HALINCDD_CSOP_HALINCDD_DIRECT/2 -> [u8_BrakeLamp]
  R_HALINCDD_CSOP_HALINCDD_DIRECT/3 -> [f32_Pedal1Vol]
  R_HALINCDD_CSOP_HALINCDD_DIRECT/4 -> [f32_Pedal2Vol]
  R_HALINCDD_CSOP_HALINCDD_DIRECT/5 -> [f32_Pedal1Ref5V]
  R_HALINCDD_CSOP_HALINCDD_DIRECT/6 -> [f32_Pedal2Ref5V]
  R_HALINCDD_CSOP_HALINCDD_DIRECT/7 -> [u8_DrDoorSW]
  R_HALINCDD_CSOP_HALINCDD_DIRECT/8 -> [u8_PsDoorSW]
  R_HALINCDD_CSOP_HALINCDD_DIRECT/9 -> [u8_RRDoorSW]
  R_HALINCDD_CSOP_HALINCDD_DIRECT/10 -> [u8_RLDoorSW]
  R_HALINCDD_CSOP_HALINCDD_DIRECT/11 -> [u8_HoodSW]
  R_HALINCDD_CSOP_HALINCDD_DIRECT/12 -> [u8_TailgateSW]
  R_HALINCDD_CSOP_HALINCDD_DIRECT/13 -> [u8_HazardSW]
  R_HALINCDD_CSOP_HALINCDD_DIRECT/14 -> [u8_SeatSW]
  R_HALINCDD_CSOP_HALINCDD_DIRECT/15 -> [u8_CrashSignal]
  R_UDSCDD_CSOP_DdmClearDTCNotification/1 -> [u8_ClearDTCcmd]
  R_HALIN_IMU_CSOP_IMUGetSixAxisVal/1 -> [s16_IMUSixAxisVal]
  R_HALIN_IMU_CSOP_IMUGetSixAxisVal/2 -> [u8_IMUSixAxisValSta]
  R_HALIN_APS_CSOP_ApsGetData/1 -> [u8_GetAPS_Progress_PCT]
  R_HALIN_APS_CSOP_ApsGetData/2 -> [u8_GetAPS_RQ_Display]
  R_HALIN_APS_CSOP_ApsGetData/3 -> [u8_GetAPS_SW_Ver]
  R_HALIN_APS_CSOP_ApsGetData/4 -> [u8_GetAPS_HW_Ver]
  R_HALIN_APS_CSOP_ApsGetData/5 -> [u8_GetAPS_ExitCondition]
  R_HALIN_APS_CSOP_ApsGetData/6 -> [f32_GetAPS_Angle_Target]
  R_HALIN_APS_CSOP_ApsGetData/7 -> [u8_GetAPS_Sta_System]
  R_HALIN_APS_CSOP_ApsGetData/8 -> [u8_GetAPS_V_Rq_EPAS_Ctrl]
  R_HALIN_APS_CSOP_ApsGetData/9 -> [u8_GetAPS_Rq_EPAS_Ctrl]
  R_HALIN_APS_CSOP_ApsGetData/10 -> [u8_GetAPS_Req]
  R_HALIN_APS_CSOP_ApsGetData/11 -> [f32_GetAPS_DecReq]
  R_HALIN_APS_CSOP_ApsGetData/12 -> [u8_GetAPS_DecReq_A]
  R_HALIN_APS_CSOP_ApsGetData/13 -> [f32_GetAPS_SpeedCmd]
  R_HALIN_APS_CSOP_ApsGetData/14 -> [u8_GetAPS_ShftPosnReq]
  R_HALIN_APS_CSOP_ApsGetData/15 -> [u8_GetAPS_VMC_Req_A]
  R_HALIN_APS_CSOP_ApsGetData/16 -> [u8_GetCAAS_Sta]
  R_HALIN_APS_CSOP_ApsGetData/17 -> [u8_GetCAAS_VMC_Req_A]
  R_HALIN_APS_CSOP_ApsGetData/18 -> [u8_GetAPS_PwrReq_cmd]
  R_HALIN_APS_CSOP_ApsGetData/19 -> [u8_GetRAPS_BCM_LockReq_Cmd]
  R_HALIN_APS_CSOP_ApsGetData/20 -> [u8_GetRAPS_BCM_Lamp_Cmd]
  R_HALIN_APS_CSOP_ApsGetData/21 -> [u8_GetRAPS_ErrWarn_Sta]
  R_HALIN_APS_CSOP_ApsGetData/22 -> [u8_GetRAPS_ErrLv1_flg]
  R_HALINCDD_CSOP_GetAcoreRebootCmd/1 -> [u8_AcoreRebootCmd]
  R_HALINCDD_CSOP_CAN1BusOff/1 -> [u8_CAN1BusOff]
  R_HALINCDD_CSOP_CAN2BusOff/1 -> [u8_CAN2BusOff]
  R_HALINCDD_CSOP_CAN3BusOff/1 -> [u8_CAN3BusOff]
  R_HALINCDD_CSOP_CAN4BusOff/1 -> [u8_CAN4BusOff]
  R_HALINCDD_CSOP_CAN5BusOff/1 -> [u8_CAN5BusOff]
  R_HALINCDD_CSOP_CAN6BusOff/1 -> [u8_CAN6BusOff]
  R_HALINCDD_CSOP_TPMSSensorIDRegGetSta/1 -> [u8_TPMSSensorIDRegSta]
  R_HALINCDD_CSOP_ReadPedalZeroPosReq/1 -> [u8_ReadPedalZeroPosReq]
  R_HALINCDD_CSOP_ResetPedalZeroPosReq/1 -> [u8_ResetPedalZeroPosReq]
  R_HALINCDD_CSOP_GetVinCode/1(Out1) -> [u8Array17_VinCode]
  [trig_Read_NVM_00] -> R_NVMReadCDD_Inner_NVM_ReadOperation/Trigger
  [trig_ReadIMUOffset_00] -> R_HALIN_IMU_CSOP_IMUGetOffsetVal/Trigger
  R_HALIN_IMU_CSOP_IMUGetOffsetVal/1(Out1) -> [s16_IMUOffsetVal]
  R_HALIN_IMU_CSOP_IMUGetOffsetVal/2(Out2) -> [u8_IMUOffsetValSta]
  [trig_GetDID] -> DIDGet_Subsystem/Trigger
  DIDGet_Subsystem/1(BHAL_DID_outputs) -> [BHAL_DID_outputs]
  Constant8/1 -> R_HALINCDD_CSOP_GetVinCode/Enable
  Mux1/1 -> [u8Array2_DKCUIDBLEVol]
  Demux/8 -> [s8_DKCUIDBLERSSI]
  Demux/4 -> [u8_DKCButton]
  Demux/1 -> Mux/1
  Demux/2 -> Mux/2
  Mux/1 -> [u8Array3_DKCData]
  Demux/7 -> Mux1/2
  Demux/5 -> [u8_DKCUIDBLEStatus]
  R_DKCData_u8Array8_DKCData_read/1 -> Demux/1
  Demux/3 -> Mux/3
  R_BHAL_CAN4_outputs_BHAL_CAN4_outputs_read/1 -> [BHAL_CAN4_outputs]
  R_BHAL_CAN2_outputs_BHAL_CAN2_outputs_read/1 -> [BHAL_CAN2_outputs]
  Demux/6 -> Mux1/1
  [u8_GetAPS_Sta_System] -> Halin_CDD/69(u8_GetAPS_Sta_System)
  hcu_main_sched/11(trig_APP_30()) -> Goto97/1
  [f32_Pedal1Vol] -> Halin_CDD/9(VHAL_AccelPedal1Vol_Raw)
  [u8Array4_HWID] -> Halin_CDD/25(u8_HWID_4byte)
  [u8_GetAPS_Req] -> Halin_CDD/72(u8_GetAPS_Req)
  [u8_CrashSignal] -> Halin_CDD/24(VHAL_CrashSignalGPIO_flg)
  [u8_RRDoorSW] -> Halin_CDD/16(VHAL_RRDoorSW_flg)
  Halin_CDD/3(BHAL_SYS_outputs) -> [BHAL_SYS_outputs]
  [u8Array9_TPMSData] -> Halin_CDD/40(TPMS_RawData)
  [u8_GetCAAS_Sta] -> Halin_CDD/78(u8_GetCAAS_Sta)
  [u8_GetAPS_VMC_Req_A] -> Halin_CDD/77(u8_GetAPS_VMC_Req_A)
  [u8Array12_ApsInUssSta] -> Halin_CDD/4(APSFaultStaData)
  From97/1 -> Halin_CDD/37(VHAL_DIDVCUKeyReadSta_flg)
  [u8_HoodSW] -> Halin_CDD/12(VHAL_HoodSW_flg)
  [u8_CurrentNMState] -> Halin_CDD/29(VHAL_CurrentNmState_enum)
  hcu_main_sched/9(trig_HAL_DKC_10_3()) -> Goto119/1
  [u32_WISR] -> Halin_CDD/54(VHAL_WisrBootReason_raw32)
  [u8_CAN5BusOff] -> Halin_CDD/61(VHAL_CAN5BusOff_raw)
  hcu_main_sched/1(trig_Read_NVM_00()) -> [trig_Read_NVM_00]
  hcu_main_sched/15(trig_HAL_OUTAFTER_50_1()) -> Goto101/1
  hcu_main_sched/14(trig_HAL_OUT_50()) -> Goto94/1
  hcu_main_sched/2(trig_ReadIMUOffset_00()) -> [trig_ReadIMUOffset_00]
  hcu_main_sched/8(trig_HAL_DKC_10_2()) -> [trig_HAL_DKC_10_2]
  [BHAL_DKC_outputs] -> P_BHAL_DKC_outputs_BHAL_DKC_outputs_write/1
  [BHAL_APM_outputs] -> P_BHAL_APM_outputs_BHAL_APM_outputs_write/1
  [BHAL_DDM_outputs] -> P_BHAL_DDM_outputs_BHAL_DDM_outputs_write/1
  [BHAL_IMU_outputs] -> P_BHAL_IMU_outputs_BHAL_IMU_outputs_write/1
  From92/1 -> Halin_CDD/38(VHAL_GetDIDVCUKey_enum)
  [u8_AcoreRebootCmd] -> Halin_CDD/56(VHAL_AcoreRebootCmd_raw)
  [u8_AlcoholPass] -> Halin_CDD/90(u8_AlcoholPass)
  [u8_CAN4BusOff] -> Halin_CDD/60(VHAL_CAN4BusOff_raw)
  [u8Array8_ApsInLevel] -> Halin_CDD/3(APSLevelData)
  [f32_GetAPS_SpeedCmd] -> Halin_CDD/75(f32_GetAPS_SpeedCmd)
  [u32_BootPath] -> Halin_CDD/87(u32_BootPath)
  [s8_AcoreReadyToSleep] -> Halin_CDD/33(VHAL_AcoreReadyToSlp_flg)
  hcu_main_sched/5(trig_GetDID()) -> [trig_GetDID]
  [u8_ApsInSysFailSta] -> Halin_CDD/7(StaFSyaIn)
  Constant5/1 -> hcu_main_sched/1(VHAL_FusionSchedReq_flg)
  [u8_IMUOffsetValSta] -> Halin_CDD/46(VHAL_IMUOffsetValSta_flg)
  hcu_main_sched/10(trig_INP_20()) -> Goto98/1
  [f32_Pedal2Ref5V] -> Halin_CDD/51(VHAL_Pedal2Ref5V_raw)
  hcu_main_sched/4(trig_GetNMID()) -> Goto106/1
  [u8Array17_VinCode] -> Halin_CDD/88(u8Array17_VinCode)
  [u8_GetRAPS_ErrLv1_flg] -> Halin_CDD/84(u8_GetRAPS_ErrLv1_flg)
  [u8_GetAPS_Progress_PCT] -> Halin_CDD/63(u8_GetAPS_Progress_PCT)
  [f32_GetAPS_Angle_Target] -> Halin_CDD/68(f32_GetAPS_Angle_Target)
  Halin_CDD/6(BHAL_IMU_outputs) -> [BHAL_IMU_outputs]
  [u8_BrakeLamp] -> Halin_CDD/21(VHAL_BrakeLampSW_flg)
  [u16Array4_ApsInDist] -> Halin_CDD/2(APSDistanceData)
  [u8_PushButton] -> Halin_CDD/89(u8_PushButton)
  hcu_main_sched/6(trig_HAL_IN_10()) -> Goto99/1
  [u8_NvmProtectSta] -> Halin_CDD/48(VHAL_NvmProtectSta_flg)
  [u8_GetAPS_ExitCondition] -> Halin_CDD/67(u8_GetAPS_ExitCondition)
  Halin_CDD/1(BHAL_APM_outputs) -> [BHAL_APM_outputs]
  hcu_main_sched/12(trig_OUTP_40()) -> Goto96/1
  [u8_TPMSDataInSta] -> Halin_CDD/39(TPMS_DataIn_flg)
  [trig_HAL_DKC_10_2] -> Subsystem/Trigger
  [u8_CAN3BusOff] -> Halin_CDD/59(VHAL_CAN3BusOff_raw)
  [BHAL_CAN4_outputs] -> Halin_CDD/42(BHAL_CAN4_outputs)
  [s16_IMUSixAxisVal] -> Halin_CDD/45(VHAL_IMUSixAxisVal_raw)
  [u8_RLDoorSW] -> Halin_CDD/17(VHAL_RLDoorSW_flg)
  [trig_HAL_CDD_10_1] -> Halin_CDD/Trigger
  [u8_GetRAPS_ErrWarn_Sta] -> Halin_CDD/83(u8_GetRAPS_ErrWarn_Sta)
  [u8_SeatSW] -> Halin_CDD/23(VHAL_SeatSW_flg)
  [u8_DrDoorSW] -> Halin_CDD/14(VHAL_DrDoorSW_flg)
  [u8_BrakeSW] -> Halin_CDD/11(VHAL_BrakeSWGPIO_flg)
  [u8_ResetPedalZeroPosReq] -> Halin_CDD/86(u8_ResetPedalZeroPosReq)
  [u8_CTDSW] -> Halin_CDD/18(VHAL_CentralDoorLockSW_flg)
  [u8_ApsInSysMode] -> Halin_CDD/8(ModOperationIn)
  [u8_CAN1BusOff] -> Halin_CDD/57(VHAL_CAN1BusOff_raw)
  From91/1 -> Halin_CDD/34(VHAL_DidXWDSta_flg)
  [u8_TailgateSW] -> Halin_CDD/13(VHAL_TailgateSW_flg)
  [u8_ApsInPASChime] -> Halin_CDD/5(ChimeIn)
  [u8_TPMSSensorIDRegSta] -> Halin_CDD/85(u8_TPMSSensorIDRegSta)
  [u8_GetRAPS_BCM_Lamp_Cmd] -> Halin_CDD/82(u8_GetRAPS_BCM_Lamp_Cmd)
  [BHAL_SYS_outputs] -> P_BHAL_SYS_outputs_BHAL_SYS_outputs_write/1
  [u8_GetAPS_SW_Ver] -> Halin_CDD/65(u8_GetAPS_SW_Ver)
  [u8_GetCAAS_VMC_Req_A] -> Halin_CDD/79(u8_GetCAAS_VMC_Req_A)
  hcu_main_sched/7(trig_HAL_CDD_10_1()) -> [trig_HAL_CDD_10_1]
  [BHAL_DID_outputs] -> Halin_CDD/55(BHAL_DIDGetData_raw)
  [u8_GetAPS_ShftPosnReq] -> Halin_CDD/76(u8_GetAPS_ShftPosnReq)
  [u8Array8_PasInDist] -> Halin_CDD/1(PASDistanceData)
  [u8_TrunkHanSW] -> Halin_CDD/22(VHAL_TrunkHanSW_flg)
  Halin_CDD/2(BHAL_GPIO_outputs) -> [BHAL_GPIO_outputs]
  [u8Array33_SWID] -> Halin_CDD/27(GetSWID_data)
  [u16_AuxBattVol100mV] -> Halin_CDD/49(VHAL_AuxBattVolmV_100mV)
  [u8_GetAPS_HW_Ver] -> Halin_CDD/66(u8_GetAPS_HW_Ver)
  [f32_Pedal2Vol] -> Halin_CDD/10(VHAL_AccelPedal2Vol_Raw)
  hcu_main_sched/13(trig_OUTP_AFTER_40_1()) -> Goto95/1
  [u8_ClearDTCcmd] -> Halin_CDD/43(VHAL_ClearDTCcmd_flg)
  [u8_GetAPS_PwrReq_cmd] -> Halin_CDD/80(u8_GetAPS_PwrReq_cmd)
  [u8_GetAPS_DecReq_A] -> Halin_CDD/74(u8_GetAPS_DecReq_A)
  [f32_GetAPS_DecReq] -> Halin_CDD/73(f32_GetAPS_DecReq)
  [u8_AnyNMID] -> Halin_CDD/28(VHAL_AnyNMID_flg)
  [u8_EvccAplusPwrUpReq] -> Halin_CDD/32(VHAL_EvccAplusPwrUpReq_flg)
  [BHAL_DID_outputs] -> P_BHAL_DID_outputs_BHAL_DID_outputs_write/1
  [u8_CAN2BusOff] -> Halin_CDD/58(VHAL_CAN2BusOff_raw)
  [BHAL_CAN2_outputs] -> Halin_CDD/41(BHAL_CAN2_outputs)
  [u8_AllowMovThdOTA] -> Halin_CDD/31(VHAL_AllowMovThd_OTA_enum)
  [s16_IMUOffsetVal] -> Halin_CDD/44(VHAL_IMUOffsetVal_raw)
  hcu_main_sched/3(trig_WDG()) -> Goto91/1
  [u8_GetAPS_V_Rq_EPAS_Ctrl] -> Halin_CDD/70(u8_GetAPS_V_Rq_EPAS_Ctrl)
  [u8_GetAPS_RQ_Display] -> Halin_CDD/64(u8_GetAPS_RQ_Display)
  [u8_GetAPS_Rq_EPAS_Ctrl] -> Halin_CDD/71(u8_GetAPS_Rq_EPAS_Ctrl)
  [BHAL_GPIO_outputs] -> P_BHAL_GPIO_outputs_BHAL_GPIO_outputs_write/1
  [u8_CAN6BusOff] -> Halin_CDD/62(VHAL_CAN6BusOff_raw)
  [u8_IMUSixAxisValSta] -> Halin_CDD/47(VHAL_IMUSixAxisValSta_flg)
  Halin_CDD/4(BHAL_TPMS_outputs) -> [BHAL_TPMS_outputs]
  [u8_BootReason] -> Halin_CDD/53(VHAL_PmicBootReason_enum)
  Halin_CDD/5(BHAL_DDM_outputs) -> [BHAL_DDM_outputs]
  [u8_HazardSW] -> Halin_CDD/20(VHAL_HazardSW_flg)
  [BHAL_TPMS_outputs] -> P_BHAL_TPMS_outputs_BHAL_TPMS_outputs_write/1
  [u8_ApsInSensorLayout] -> Halin_CDD/6(SNSRLayoutIn)
  From96/1 -> Halin_CDD/35(VHAL_DidXWDData_enum)
  Constant6/1 -> Halin_CDD/26(GetSWID_status)
  [u8_GetRAPS_BCM_LockReq_Cmd] -> Halin_CDD/81(u8_GetRAPS_BCM_LockReq_Cmd)
  [u8Array1024_NvmReadArray] -> Halin_CDD/36(HAL_NvmReadData_raw)
  [f32_Pedal1Ref5V] -> Halin_CDD/50(VHAL_Pedal1Ref5V_raw)
  [u8_PsDoorSW] -> Halin_CDD/15(VHAL_PsDoorSW_flg)
  [VHAL_NetworkReqCalled_flg] -> Halin_CDD/52(VHAL_NetworkReqCalled_flg)
  [u8_PwrReqOTA] -> Halin_CDD/30(VHAL_PwrReq_OTA_enum)
  Halin_CDD/7(Enable_decrypt) -> Subsystem/1(Enable_Decrypt)
  Halin_CDD/8(AESKey) -> Subsystem/2(In2)
  Halin_CDD/9(DKCRawData) -> Subsystem/3(In3)
  [BHAL_CAN4_outputs] -> Subsystem/4(BHAL_CAN4_outputs)
  [u8Array3_DKCData] -> Subsystem/5(u8Array3_DKCData)
  [u8_DKCButton] -> Subsystem/6(u8_DKCButton)
  [u8_DKCUIDBLEStatus] -> Subsystem/7(u8_DKCUIDBLEStatus)
  [u8Array2_DKCUIDBLEVol] -> Subsystem/8(u8Array2_DKCUIDBLEVol)
  [s8_DKCUIDBLERSSI] -> Subsystem/9(s8_DKCUIDBLERSSI)
  Subsystem/1(BHAL_DKC_outputs) -> [BHAL_DKC_outputs]
  Ground_1/1 -> Halin_CDD/19(VHAL_CentralDoorUnLockSW_flg)
  [u8_BmsAplus] -> Halin_CDD/91(u8_BmsAplus)
  IRV_u8_BMSAplus_read/1 -> [u8_BmsAplus]
